simulink model "AFE_2L_H4Q"  (R2013b)
settings: Solver=FixedStepDiscrete  SolverMode=SingleTasking  StartTime=0.0  StopTime=0.9  FixedStep=Tpas  RelTol=1e-3
values from neighbouring files (symbols this model uses):
  Cbus = 330e-3    (= 0.33)    [AFE_FV_Params.m]    (also in AFE_FV_ParamsPV4.m; Params.m)
  fmod4Q = 1e3    (= 1000)    [AFE_FV_Params.m]    (also in AFE_FV_ParamsPV4.m; Params.m)
  Freq = 50    [AFE_FV_Params.m]    (also in AFE_FV_ParamsPV4.m; Params.m)
  hys = 450    [AFE_FV_Params.m]    (also in AFE_FV_ParamsPV4.m; Params.m = 300)
  I4Q = 1/0.02    (= 50)    [AFE_FV_Params.m]    (also in AFE_FV_ParamsPV4.m = (P4Q+Numd(2)/Dend(1))/Ts; CalcPIAndFilters.m = (P4Q+Numd(2)/Dend(1))/Ts; Params.m = (P4Q+Numd(2)/Dend(1))/Ts)
  Kac = 1/(Vac*sqrt(2/3))    [AFE_FV_Params.m]    (also in AFE_FV_ParamsPV4.m; Params.m)
  KLP4Q = 0.01    [AFE_FV_Params.m]    (also in AFE_FV_ParamsPV4.m = NLPripd(2); CalcPIAndFilters.m = NLPripd(2); Params.m = NLPripd(2))
  L = .1    (= 0.1)    [AFE_FV_Params.m]    (also in AFE_FV_ParamsPV4.m; Params.m)
  Lac = 8.1487e-04    (= 0.00081487)    [AFE_FV_Params.m]    (also in AFE_FV_ParamsPV4.m; Params.m)
  P4Q = 0.071    [AFE_FV_Params.m]    (also in AFE_FV_ParamsPV4.m = Numd(1)/Dend(1); CalcPIAndFilters.m = Numd(1)/Dend(1); Params.m = Numd(1)/Dend(1))
  R = .28    (= 0.28)    [AFE_FV_Params.m]    (also in AFE_FV_ParamsPV4.m; Params.m)
  SatPIH4Q = .95    (= 0.95)    [AFE_FV_Params.m]    (also in AFE_FV_ParamsPV4.m; Params.m)
  Satv = 1500    [AFE_FV_Params.m]    (also in AFE_FV_ParamsPV4.m; Params.m = 3.6e6*sqrt(2)/(sqrt(3)*Vac))
  TLP4Q = -0.99    [AFE_FV_Params.m]    (also in AFE_FV_ParamsPV4.m = DLPripd(2); CalcPIAndFilters.m = DLPripd(2); Params.m = DLPripd(2))
  Tpas = 10e-6    (= 1e-05)    [AFE_FV_Params.m]    (also in AFE_FV_ParamsPV4.m; Params.m)
  Vac = 2000    [AFE_FV_Params.m]    (also in AFE_FV_ParamsPV4.m; Params.m)
  Vdc = 5000    [AFE_FV_Params.m]    (also in AFE_FV_ParamsPV4.m; Params.m)
undefined symbols (not defined in the file or in its folder): Rac
libraries: powerlib x27, powerlib_meascontrol x17, simulink x14
settings Model: Creator=LiberT  LastModifiedBy=LiberT
settings DataIOCC: SignalLoggingSaveFormat=ModelDataLogs
settings OptimizationCC: ExpressionDepthLimit=2147483647
settings DebuggingCC: MultiTaskDSMMsg=warning  MultiTaskCondExecSysMsg=none  FcnCallInpInsideContextMsg=EnableAllAsWarning  StateNameClashWarn=warning
settings RTWCC: IncludeERTFirstTime=on

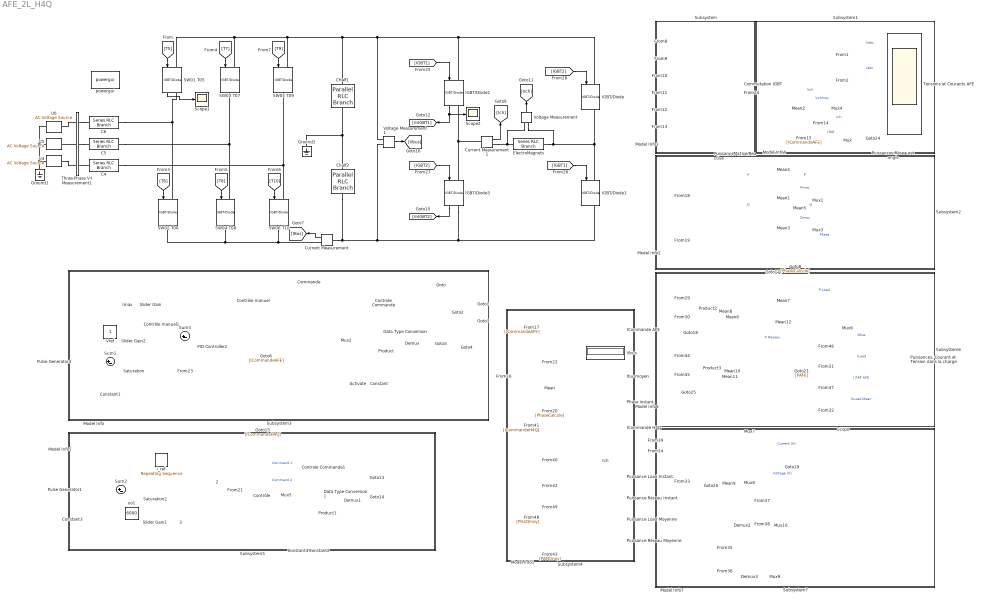
== system AFE_2L_H4Q ==
  " 2" : ManualSwitch
  " 3" : ManualSwitch  CurrentSetting=0
  Activate : Constant  Value=0
  C4 : powerlib/Elements/Series RLC Branch  LConnTagsString=__new0  RConnTagsString=__new0  BranchType=L  Resistance=Rac  Inductance=Lac  SetiL0=off  InitialCurrent=0  Capacitance=300e-3  Setx0=off  InitialVoltage=0  Measurements=None
  C5 : powerlib/Elements/Series RLC Branch  LConnTagsString=__new0  RConnTagsString=__new0  BranchType=L  Resistance=Rac  Inductance=Lac  SetiL0=off  InitialCurrent=0  Capacitance=300e-3  Setx0=off  InitialVoltage=0  Measurements=None
  C6 : powerlib/Elements/Series RLC Branch  LConnTagsString=__new0  RConnTagsString=__new0  BranchType=L  Resistance=Rac  Inductance=Lac  SetiL0=off  InitialCurrent=0  Capacitance=300e-3  Setx0=off  InitialVoltage=0  Measurements=None
  CHalf1 : powerlib/Elements/Parallel RLC Branch  LConnTagsString=a  RConnTagsString=__new0  BranchType=C  Resistance=inf  Inductance=inf  SetiL0=off  InitialCurrent=0  Capacitance=Cbus*2  Setx0=on  InitialVoltage=Vdc/2  Measurements=Branch voltage
  Chalf2 : powerlib/Elements/Parallel RLC Branch  LConnTagsString=a  RConnTagsString=__new0  BranchType=C  Resistance=inf  Inductance=inf  SetiL0=off  InitialCurrent=0  Capacitance=Cbus*2  Setx0=on  InitialVoltage=Vdc/2  Measurements=Branch voltage
  Commande : Subsystem
  Commutation IGBT : Scope  NumInputPorts=6
      settings: TickLabels=on  TimeRange=0.04  YMin=-0.2~-0.2~-0.2~-0.2~-0.2~-0.2  YMax=1.2~1.2~1.2~1.2~1.2~1.2
  Constant : Constant  Value=[1 1 1 1 1 1]
  Constant1 : Constant  Value=6000
  Constant2 : Constant  Value=[1 1]
  Constant3 : Constant  Value=6000
  Constant4 : Constant  Value=0
  Controle Commande : ManualSwitch
  Controle Commande1 : ManualSwitch
  Contrôle : Subsystem  TreatAsAtomicUnit=on
      settings: MinAlgLoopOccurrences=on
  Contrôle manuel : ManualSwitch  CurrentSetting=0
  Contrôle manuel1 : ManualSwitch
  Current Measurement : powerlib/Measurements/Current Measurement  PhasorSimulation=off  OutputType=Complex  PSBequivalent=0
  Current Measurement1 : powerlib/Measurements/Current Measurement  PhasorSimulation=off  OutputType=Complex  PSBequivalent=0
  Data Type Conversion : DataTypeConversion  OutDataTypeStr=boolean
  Data Type Conversion1 : DataTypeConversion  OutDataTypeStr=boolean
  Demux : Demux  Outputs=6
  Demux1 : Demux  Outputs=2
  Demux2 : Demux  Outputs=2
  Demux3 : Demux  Outputs=2
  "ElectroMagnets " : powerlib/Elements/Series RLC Branch  LConnTagsString=__new0  RConnTagsString=__new0  BranchType=RL  Resistance=R  Inductance=L  SetiL0=off  InitialCurrent=0  Capacitance=1e-6  Setx0=off  InitialVoltage=0  Measurements=Branch voltage and current
  Ground1 : powerlib/Elements/Ground  LConnTagsString=a
  Ground2 : powerlib/Elements/Ground  LConnTagsString=a
  "ICommande AFE " : Display
  ICommande H4Q : Display
  IGBT/Diode{,1..3} (4 alike) : powerlib/Power Electronics/IGBT//Diode  Ron=1e-3  Rs=1e5  Cs=inf  Measurements=on
  Ibusmoyen : Display
  Ich : Display
  Imax : Constant  Value=5000
  Mean{,1..3} (4 alike) : powerlib_meascontrol/Measurements/Mean  Freq=50  Vinit=0  Ts=Tpas
  Mean10 : powerlib_meascontrol/Measurements/Mean  Freq=fmod4Q/2  Vinit=0  Ts=Tpas
  Mean11 : powerlib_meascontrol/Measurements/Mean  Freq=1/.9  Vinit=0  Ts=Tpas
  Mean12 : powerlib_meascontrol/Measurements/Mean  Freq=fmod4Q  Vinit=0  Ts=Tpas
  Mean4 : powerlib_meascontrol/Measurements/Mean  Freq=fmod4Q*3  Vinit=0  Ts=Tpas
  Mean5 : powerlib_meascontrol/Measurements/Mean  Freq=fmod4Q*3  Vinit=0  Ts=Tpas
  Mean6 : powerlib_meascontrol/Measurements/Mean  Freq=1/.9  Vinit=0  Ts=Tpas
  Mean7 : powerlib_meascontrol/Measurements/Mean  Freq=fmod4Q  Vinit=0  Ts=Tpas
  Mean8 : powerlib_meascontrol/Measurements/Mean  Freq=fmod4Q/2  Vinit=0  Ts=Tpas
  Mean9 : powerlib_meascontrol/Measurements/Mean  Freq=fmod4Q  Vinit=0  Ts=Tpas
  Model Info : simulink/Model-Wide Utilities/Model Info  InitialBlockCM=None  BlockCM=None  Frame=on  DisplayStringWithTags=Commande AFE  HorizontalTextAlignment=Center  LeftAlignmentValue=0.5  SourceBlockDiagram=AFE_2L_H4Q  TagMaxNumber=20
  Model Info{1..4,6..7} (6 alike) : simulink/Model-Wide Utilities/Model Info  InitialBlockCM=None  BlockCM=None  Frame=on  DisplayStringWithTags=Résultats  HorizontalTextAlignment=Center  LeftAlignmentValue=0.5  SourceBlockDiagram=AFE_2L_H4Q  TagMaxNumber=20
  Model Info5 : simulink/Model-Wide Utilities/Model Info  InitialBlockCM=None  BlockCM=None  Frame=on  DisplayStringWithTags=Commande H4Q  HorizontalTextAlignment=Center  LeftAlignmentValue=0.5  SourceBlockDiagram=AFE_2L_H4Q  TagMaxNumber=20
  Mux{,1,3..10} (10 alike) : Mux  Inputs=2
  Mux2 : Mux  Inputs=6
  PID Controller2 : simulink/Continuous/PID Controller  Controller=PI  TimeDomain=Discrete-time  SampleTime=Tpas  IntegratorMethod=Forward Euler  FilterMethod=Forward Euler  Form=Parallel  P=150  I=1.2e4  D=0  N=100  InitialConditionSource=internal  InitialConditionForIntegrator=0  InitialConditionForFilter=0  ExternalReset=none  LimitOutput=on  UpperSaturationLimit=Satv  LowerSaturationLimit=-Satv  LinearizeAsGain=on  AntiWindupMode=clamping  Kb=1  TrackingMode=off  Kt=1  PParamMin=[]  PParamMax=[]  IParamMin=[]  IParamMax=[]  DParamMin=[]  DParamMax=[]  NParamMin=[]  NParamMax=[]  KbParamMin=[]  KbParamMax=[]  KtParamMin=[]  KtParamMax=[]  POutMin=[]  POutMax=[]  IOutMin=[]  IOutMax=[]  DOutMin=[]  DOutMax=[]  NOutMin=[]  NOutMax=[]  KbOutMin=[]  KbOutMax=[]  KtOutMin=[]  KtOutMax=[]  IntegratorOutMin=[]  IntegratorOutMax=[]  FilterOutMin=[]  FilterOutMax=[]  SumOutMin=[]  SumOutMax=[]  SumI1OutMin=[]  SumI1OutMax=[]  SumI2OutMin=[]  SumI2OutMax=[]  SumI3OutMin=[]  SumI3OutMax=[]  SumDOutMin=[]  SumDOutMax=[]  SaturationOutMin=[]  SaturationOutMax=[]  IntegratorContinuousStateAttributes=''  IntegratorStateMustResolveToSignalObject=off  IntegratorRTWStateStorageClass=Auto  FilterContinuousStateAttributes=''  FilterStateMustResolveToSignalObject=off  FilterRTWStateStorageClass=Auto
  Phase instant. : Display
  Product{,1..3} (4 alike) : Product
  Puissance Active/Reactive : Subsystem
  Puissance Load Instant. : Display
  Puissance Load Moyenne : Display
  Puissance Réseau Instant : Display
  Puissance Réseau Moyenne : Display
  Puissances Réseau et angle : Scope  NumInputPorts=3
      settings: TickLabels=on  TimeRange=0.04  YMin=-1000000~-400000~-200  YMax=10000000~350000~200  SaveName=ScopeData2
  "Puissances, Courant et Tension dans la charge" : Scope  NumInputPorts=5
      settings: TickLabels=on  ShowLegends=on  TimeRange=0.9  YMin=-20000000~3000~-1000~-3000~-5000  YMax=20000000~5250~7000~3000~5000  SaveName=ScopeData3
  Pulse Generator1 : DiscretePulseGenerator  Amplitude=12000  Period=floor(.4 /Tpas)  PulseWidth=floor(.4 * .5 / Tpas)  PhaseDelay=floor(.001 / Tpas)  SampleTime=Tpas
  Pulse Generator3 : DiscretePulseGenerator  Amplitude=12000  Period=floor(.2/Tpas)  PulseWidth=floor(.2/2/Tpas)  SampleTime=Tpas
  SW01 T05 : powerlib/Power Electronics/IGBT//Diode  Ron=1e-3  Rs=1e5  Cs=Tpas  Measurements=on
  SW02 T06 : powerlib/Power Electronics/IGBT//Diode  Ron=1e-3  Rs=1e5  Cs=Tpas  Measurements=off
  SW03 T07 : powerlib/Power Electronics/IGBT//Diode  Ron=1e-3  Rs=1e5  Cs=Tpas  Measurements=off
  SW04 T08 : powerlib/Power Electronics/IGBT//Diode  Ron=1e-3  Rs=1e5  Cs=Tpas  Measurements=off
  SW05 T09 : powerlib/Power Electronics/IGBT//Diode  Ron=1e-3  Rs=1e5  Cs=Tpas  Measurements=off
  SW06 T10 : powerlib/Power Electronics/IGBT//Diode  Ron=1e-3  Rs=1e5  Cs=Tpas  Measurements=off
  Saturation : Saturate  UpperLimit=5100  LowerLimit=5000
  Saturation2 : Saturate  UpperLimit=5000  LowerLimit=2000
  Scope : Scope  NumInputPorts=6
      settings: TimeRange=0.9  YMin=-7000~-12500~-0.1~-0.1~-7000~-6000  YMax=7000~7500~1.1~1.1~7000~6000  SaveName=hash  MaxDataPoints=10000
  Scope1 : Scope
      settings: SaveName=IGBTA
  Scope2 : Scope
      settings: SaveName=IGBTH
  Slider Gain : simulink/Math Operations/Slider Gain  low=0  gain=0.22  high=1
  Slider Gain1 : simulink/Math Operations/Slider Gain  low=0  gain=0.54  high=1
  Slider Gain2 : simulink/Math Operations/Slider Gain  low=0  gain=5000  high=6000
  Subsystem : Subsystem
      mask Display: disp('')
  Subsystem1 : Subsystem
      mask Display: disp('')
  Subsystem2 : Subsystem
      mask Display: disp('')
  Subsystem3 : Subsystem
      mask Display: disp('')
  Subsystem4 : Subsystem
      mask Display: disp('')
  Subsystem5 : Subsystem
      mask Display: disp('')
  Subsystem6 : Subsystem
      mask Display: disp('')
  Subsystem7 : Subsystem
      mask Display: disp('')
  Sum1 : Sum  Inputs=|+-
  Sum2 : Sum  Inputs=|+-
  Sum3 : Sum  Inputs=|+-
  Tensions et Courants AFE : Scope  NumInputPorts=4
      settings: TickLabels=on  ShowLegends=on  TimeRange=0.04  YMin=-1750~-2000~3000~-2000  YMax=1750~2000~5150~2000  SaveName=hach4quadrants
  Three-Phase V-I Measurement1 : powerlib/Measurements/Three-Phase V-I Measurement  VoltageMeasurement=phase-to-ground  SetLabelV=on  LabelV=Vabc  Vpu=off  VpuLL=off  CurrentMeasurement=yes  SetLabelI=on  LabelI=Iabc  Ipu=off  Pbase=100e6  Vbase=500e3  OutputType=Complex  PhasorSimulation=off  PSBequivalent=0
  U4 : powerlib/Electrical Sources/AC Voltage Source  Amplitude=Vac*sqrt(2/3)  Phase=120  Frequency=Freq  SampleTime=Tpas  Measurements=Voltage
  U5 : powerlib/Electrical Sources/AC Voltage Source  Amplitude=Vac*sqrt(2/3)  Phase=-120  Frequency=Freq  SampleTime=Tpas  Measurements=Voltage
  U6 : powerlib/Electrical Sources/AC Voltage Source  Amplitude=Vac*sqrt(2/3)  Phase=0  Frequency=Freq  SampleTime=Tpas  Measurements=Voltage
  Vbus : Display
  Voltage Measurement : powerlib/Measurements/Voltage Measurement  PhasorSimulation=off  OutputType=Complex  PSBequivalent=0
  Voltage Measurement1 : powerlib/Measurements/Voltage Measurement  PhasorSimulation=off  OutputType=Complex  PSBequivalent=0
  Vref : Constant  SampleTime=Tpas
  "i_ref " : simulink/Sources/Repeating Sequence  rep_seq_t="[0 108.51e-3 127.6e-3 132e-3 200e-3 250e-3 283.33e-3 310e-3 366.66e-3  490e-3 533e-3 683.33e-3 900e-3]"  rep_seq_y=[333 333 1000 1031 1500 2000 2500 3000 4000 6000 6000 333 333]
  powergui : powerlib/powergui  Priority=1  SimulationMode=Discrete  SolverType=Tustin  SampleTime=Tpas  frequency=60  SPID=off  DisableSnubberDevices=off  DisableRonSwitches=off  DisableVfSwitches=off  SwTol=0  Interpol=off  DisplayEquations=off  frequencyindice=50  Pbase=100e6  ErrMax=1e-4  Iterations=50  UnitsV=kV  UnitsW=MW  FunctionMessages=off  echomessages=off  HookPort=off  EnableUseOfTLC=off  x0status=blocks  RestoreLinks=warning  ResistiveCurrentMeasurement=off  Frange=[0:2:500]  Ylog=off  Xlog=on  ShowGrid=off  save=off  variable=ZData  structure=ScopeData1  ZoomFFT=off  StartTime=18  cycles=100  DisplayStyle=1  fundamental=50  FreqAxis=off  MaxFrequency=2000  frequencyindicesteady=1  RmsSteady=1  display=off  Ts=0  methode=off
  uo1 : Constant  Value=6000
  wires:
  [T5] -> SW01 T05/1
  Current Measurement/1 -> [IBus]
  [T7] -> SW03 T07/1
  [T9] -> SW05 T09/1
  [T10] -> SW06 T10/1
  [T8] -> SW04 T08/1
  [T6] -> SW02 T06/1
  [T5] -> Commutation IGBT/1
  [T6] -> Commutation IGBT/2
  [T7] -> Commutation IGBT/3
  [T8] -> Commutation IGBT/4
  [T9] -> Commutation IGBT/5
  [T10] -> Commutation IGBT/6
  [Vabc] -> Tensions et Courants AFE/1  "Vabc"
  [Iabc] -> Tensions et Courants AFE/2  "Iabc"
  Imax/1 -> Slider Gain/1
  [IBus] -> Mux/1  "Ich"
  [ICommandeAFE] -> Mux/2  "I Ref"
  Mux/1 -> [IBusScope], Tensions et Courants AFE/4
  Mean/1 -> Ibusmoyen/1
  [Vbus] -> Vbus/1
  [IBus] -> Mean/1
  [ICommandeAFE] -> "ICommande AFE "/1
  [Vbus] -> Sum3/2
  Vref/1 -> Slider Gain2/1
  Sum3/1 -> PID Controller2/1
  Constant/1 -> Product/2
  Activate/1 -> Product/1
  Commande/1(T5) -> Mux2/1
  Commande/2(T6) -> Mux2/2
  Commande/3(T7) -> Mux2/3
  Commande/4(T8) -> Mux2/4
  Commande/5(T9) -> Mux2/5
  Commande/6(T10) -> Mux2/6
  Controle Commande/1 -> Demux/1
  Mux2/1 -> Controle Commande/1
  Demux/1 -> [T5]
  Demux/2 -> [T6]
  Demux/3 -> [T7]
  Demux/4 -> [T8]
  Demux/5 -> [T9]
  Demux/6 -> [T10]
  [Vabc] -> Puissance Active/Reactive/1(Vabc)
  [Iabc] -> Puissance Active/Reactive/2(Iabc)
  Puissance Active/Reactive/1(P) -> Mean4/1, Mean1/1  "P"
  Puissance Active/Reactive/2(Q) -> Mean3/1, Mean5/1  "Q"
  Puissance Active/Reactive/3(PhC) -> Puissances Réseau et angle/3, [PhaseCalcule]  "Phase"
  Mean1/1 -> Mux1/2  "Pmoy"
  Mux1/1 -> Puissances Réseau et angle/1
  Mean3/1 -> Mux3/2  "Qmoy"
  Mux3/1 -> Puissances Réseau et angle/2
  Mux4/1 -> Tensions et Courants AFE/3
  [Vbus] -> Mux4/1, Mean2/1  "Vch"
  Mean2/1 -> Mux4/2  "Vchmoy"
  [PhaseCalcule] -> Phase instant./1
  PID Controller2/1 -> Contrôle manuel/2
  Slider Gain/1 -> Contrôle manuel/1
  Contrôle manuel/1 -> Commande/1(In1), [ICommandeAFE]
  Data Type Conversion/1 -> Controle Commande/2
  Product/1 -> Data Type Conversion/1
  Sum1/1 -> Saturation/1
  Pulse Generator3/1 -> Sum1/1
  Constant1/1 -> Sum1/2
  Contrôle manuel1/1 -> Sum3/1
  Slider Gain2/1 -> Contrôle manuel1/1
  Saturation/1 -> Contrôle manuel1/2
  IGBT/Diode2/1 -> Scope2/1, [mIGBT1]
  IGBT/Diode3/1 -> [mIGBT2]
  [IGBT1] -> IGBT/Diode2/1
  [IGBT1] -> IGBT/Diode1/1
  [IGBT2] -> IGBT/Diode3/1
  [IGBT2] -> IGBT/Diode/1
  Current Measurement1/1 -> [Ich]
  Voltage Measurement/1 -> [Vch]
  Constant2/1 -> Product1/2
  Constant4/1 -> Product1/1
  Controle Commande1/1 -> Demux1/1
  Mux5/1 -> Controle Commande1/1
  Demux1/1 -> [IGBT1]
  Demux1/2 -> [IGBT2]
  Data Type Conversion1/1 -> Controle Commande1/2
  Product1/1 -> Data Type Conversion1/1
  " 2"/1 -> [ICommandeH4Q], Contrôle/1(Iref)
  [Ich] -> Contrôle/2(IL)
  Contrôle/2(C2) -> Mux5/2  "Command 2"
  Contrôle/1(C1) -> Mux5/1  "Command 1"
  uo1/1 -> Slider Gain1/1
  Slider Gain1/1 -> " 3"/2
  Saturation2/1 -> " 3"/1
  Constant3/1 -> Sum2/2
  "i_ref "/1 -> " 2"/1
  " 3"/1 -> " 2"/2
  Pulse Generator1/1 -> Sum2/1
  Sum2/1 -> Saturation2/1
  Voltage Measurement1/1 -> [Vbus]
  Mean4/1 -> Mux1/1  "P"
  Mean5/1 -> Mux3/1  "Q"
  Mean6/1 -> [PH4Qmoy]
  [Vch] -> Product2/1
  [Ich] -> Product2/2
  Product2/1 -> Mean8/1
  Mean8/1 -> Mean6/1, Mean7/1
  Mux7/1 -> [ILoadScope], Scope/1  "Current (A)"
  Mux8/1 -> Scope/2  "Voltage (V)"
  [Ich] -> Mux7/2
  [mIGBT1] -> Demux2/1
  Mean9/1 -> [VMeanLoad], Mux8/2
  [Vch] -> Mux8/1, Mean9/1
  [mIGBT2] -> Demux3/1
  [IGBT1] -> Scope/3
  Mux9/1 -> Scope/6
  Mux10/1 -> Scope/5
  [IGBT2] -> Scope/4
  Demux2/1 -> Mux10/1
  Demux3/1 -> Mux10/2
  Demux2/2 -> Mux9/1
  Demux3/2 -> Mux9/2
  [ICommandeH4Q] -> Mux7/1
  [PAFEmoy] -> Puissance Réseau Moyenne/1
  [PH4Q] -> Puissance Load Instant./1
  [Ich] -> Ich/1
  [ICommandeH4Q] -> ICommande H4Q/1
  Mean7/1 -> [PH4Q], Mux6/1  "P Load"
  [VMeanLoad] -> "Puissances, Courant et Tension dans la charge"/5  "VLoad Mean"
  Mux6/1 -> "Puissances, Courant et Tension dans la charge"/1
  [Vbus] -> "Puissances, Courant et Tension dans la charge"/2  "VBus"
  [ILoadScope] -> "Puissances, Courant et Tension dans la charge"/3  "ILoad"
  [ICommandeAFE] -> "Puissances, Courant et Tension dans la charge"/4  "I REF AFE"
  [IBus] -> Product3/1
  [Vbus] -> Product3/2
  Product3/1 -> Mean10/1
  Mean10/1 -> Mean11/1, Mean12/1  "P Réseau"
  Mean11/1 -> [PAFEmoy]
  [PAFE] -> Puissance Réseau Instant/1
  [PH4Qmoy] -> Puissance Load Moyenne/1
  Mean12/1 -> [PAFE], Mux6/2
  SW01 T05/1 -> Scope1/1
  connections:
  Current Measurement/RConn1 -- SW06 T10/RConn1 -- SW04 T08/RConn1 -- SW02 T06/RConn1
  SW02 T06/LConn1 -- C6/LConn1 -- SW01 T05/RConn1
  SW06 T10/LConn1 -- C4/LConn1 -- SW05 T09/RConn1
  SW04 T08/LConn1 -- C5/LConn1 -- SW03 T07/RConn1
  Three-Phase V-I Measurement1/LConn1 -- C6/RConn1
  Three-Phase V-I Measurement1/RConn1 -- U6/RConn1
  Three-Phase V-I Measurement1/RConn2 -- U5/RConn1
  Three-Phase V-I Measurement1/LConn2 -- C5/RConn1
  C4/RConn1 -- Three-Phase V-I Measurement1/LConn3
  U4/RConn1 -- Three-Phase V-I Measurement1/RConn3
  IGBT/Diode3/RConn1 -- Voltage Measurement1/LConn2 -- Chalf2/RConn1 -- Current Measurement/LConn1 -- IGBT/Diode1/RConn1
  U4/LConn1 -- U6/LConn1 -- U5/LConn1 -- Ground1/LConn1
  Chalf2/LConn1 -- Ground2/LConn1 -- CHalf1/RConn1
  IGBT/Diode3/LConn1 -- Current Measurement1/LConn1 -- IGBT/Diode2/RConn1
  SW01 T05/LConn1 -- Voltage Measurement1/LConn1 -- IGBT/Diode2/LConn1 -- IGBT/Diode/LConn1 -- CHalf1/LConn1 -- SW05 T09/LConn1 -- SW03 T07/LConn1
  "ElectroMagnets "/RConn1 -- Voltage Measurement/LConn2 -- IGBT/Diode1/LConn1 -- IGBT/Diode/RConn1
  Current Measurement1/RConn1 -- Voltage Measurement/LConn1 -- "ElectroMagnets "/LConn1

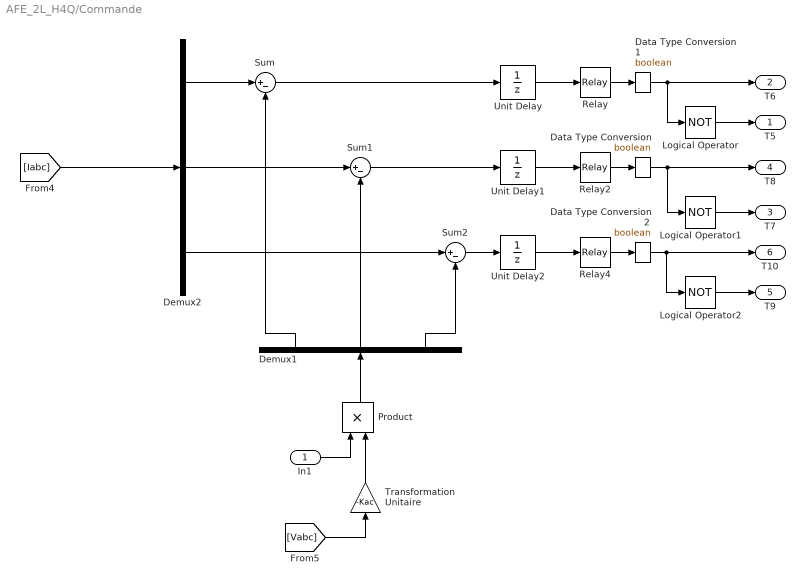
== system AFE_2L_H4Q/Commande ==
  In1 : Inport
  Data Type Conversion : DataTypeConversion  OutDataTypeStr=boolean
  Data Type Conversion1 : DataTypeConversion  OutDataTypeStr=boolean
  Data Type Conversion2 : DataTypeConversion  OutDataTypeStr=boolean
  Demux1 : Demux  Outputs=3
  Demux2 : Demux  Outputs=3
  Logical Operator : Logic  Operator=NOT  AllPortsSameDT=off
  Logical Operator1 : Logic  Operator=NOT  AllPortsSameDT=off
  Logical Operator2 : Logic  Operator=NOT  AllPortsSameDT=off
  Product : Product
  Relay : Relay  OnSwitchValue=hys  OffSwitchValue=-hys
  Relay2 : Relay  OnSwitchValue=hys  OffSwitchValue=-hys
  Relay4 : Relay  OnSwitchValue=hys  OffSwitchValue=-hys
  Sum : Sum  Inputs=|+-
  Sum1 : Sum  Inputs=|+-
  Sum2 : Sum  Inputs=|+-
  Transformation Unitaire : Gain  Gain=-Kac
  Unit Delay : UnitDelay  SampleTime=-1
  Unit Delay1 : UnitDelay  SampleTime=-1
  Unit Delay2 : UnitDelay  SampleTime=-1
  T5 : Outport
  T6 : Outport  Port=2
  T7 : Outport  Port=3
  T8 : Outport  Port=4
  T9 : Outport  Port=5
  T10 : Outport  Port=6
  wires:
  Demux2/1 -> Sum/1
  Demux2/2 -> Sum1/1
  Demux2/3 -> Sum2/1
  Sum/1 -> Unit Delay/1
  Sum1/1 -> Unit Delay1/1
  Sum2/1 -> Unit Delay2/1
  Unit Delay/1 -> Relay/1
  Unit Delay1/1 -> Relay2/1
  Unit Delay2/1 -> Relay4/1
  Logical Operator/1 -> T5/1
  Logical Operator1/1 -> T7/1
  Logical Operator2/1 -> T9/1
  Relay/1 -> Data Type Conversion1/1
  Relay2/1 -> Data Type Conversion/1
  Relay4/1 -> Data Type Conversion2/1
  [Iabc] -> Demux2/1
  [Vabc] -> Transformation Unitaire/1
  Demux1/1 -> Sum/2
  Demux1/2 -> Sum1/2
  Demux1/3 -> Sum2/2
  Data Type Conversion/1 -> T8/1, Logical Operator1/1
  Data Type Conversion1/1 -> T6/1, Logical Operator/1
  Data Type Conversion2/1 -> T10/1, Logical Operator2/1
  Transformation Unitaire/1 -> Product/2
  In1/1 -> Product/1
  Product/1 -> Demux1/1

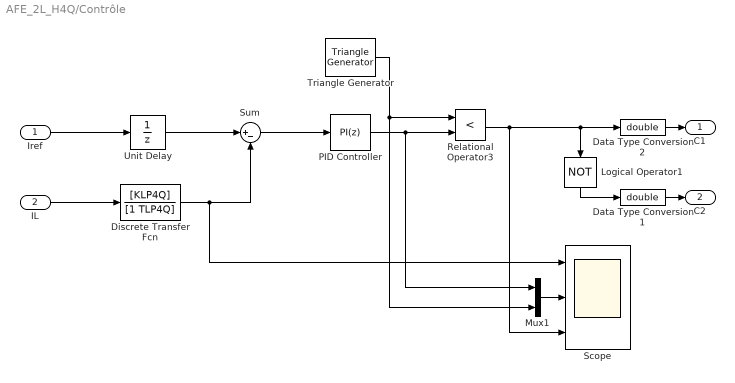
== system AFE_2L_H4Q/Contrôle ==
  Iref : Inport
  IL : Inport  Port=2
  Data Type Conversion1 : DataTypeConversion  OutDataTypeStr=double
  Data Type Conversion2 : DataTypeConversion  OutDataTypeStr=double
  Discrete Transfer Fcn : DiscreteTransferFcn  Numerator=[KLP4Q]  Denominator=[1 TLP4Q]
  Logical Operator1 : Logic  Operator=NOT  AllPortsSameDT=off  OutDataTypeStr=boolean
  Mux1 : Mux  Inputs=2
  PID Controller : simulink/Continuous/PID Controller  Controller=PI  TimeDomain=Discrete-time  SampleTime=Tpas  IntegratorMethod=Forward Euler  FilterMethod=Forward Euler  Form=Parallel  P=P4Q  I=I4Q  D=0  N=100  InitialConditionSource=internal  InitialConditionForIntegrator=0  InitialConditionForFilter=0  ExternalReset=none  LimitOutput=on  UpperSaturationLimit=SatPIH4Q  LowerSaturationLimit=-SatPIH4Q  LinearizeAsGain=on  AntiWindupMode=clamping  Kb=1  TrackingMode=off  Kt=1  PParamMin=[]  PParamMax=[]  IParamMin=[]  IParamMax=[]  DParamMin=[]  DParamMax=[]  NParamMin=[]  NParamMax=[]  KbParamMin=[]  KbParamMax=[]  KtParamMin=[]  KtParamMax=[]  POutMin=[]  POutMax=[]  IOutMin=[]  IOutMax=[]  DOutMin=[]  DOutMax=[]  NOutMin=[]  NOutMax=[]  KbOutMin=[]  KbOutMax=[]  KtOutMin=[]  KtOutMax=[]  IntegratorOutMin=[]  IntegratorOutMax=[]  FilterOutMin=[]  FilterOutMax=[]  SumOutMin=[]  SumOutMax=[]  SumI1OutMin=[]  SumI1OutMax=[]  SumI2OutMin=[]  SumI2OutMax=[]  SumI3OutMin=[]  SumI3OutMax=[]  SumDOutMin=[]  SumDOutMax=[]  SaturationOutMin=[]  SaturationOutMax=[]  IntegratorContinuousStateAttributes=''  IntegratorStateMustResolveToSignalObject=off  IntegratorRTWStateStorageClass=Auto  FilterContinuousStateAttributes=''  FilterStateMustResolveToSignalObject=off  FilterRTWStateStorageClass=Auto
  Relational Operator3 : RelationalOperator  Operator=<  OutDataTypeStr=boolean
  Scope : Scope  NumInputPorts=3
      settings: TimeRange=0.01  YMin=0~-1.2~-5  YMax=6000~1.2~5
  Sum : Sum  Inputs=|+-
  Triangle Generator : powerlib_meascontrol/Pulse & Signal Generators/Triangle Generator  Freq=fmod4Q  Phase=180  Ts=Tpas
  Unit Delay : UnitDelay  SampleTime=-1
  C1 : Outport
  C2 : Outport  Port=2
  wires:
  Triangle Generator/1 -> Mux1/2, Relational Operator3/1
  Relational Operator3/1 -> Logical Operator1/1, Data Type Conversion2/1, Scope/3
  Data Type Conversion2/1 -> C1/1
  Logical Operator1/1 -> Data Type Conversion1/1
  Data Type Conversion1/1 -> C2/1
  Discrete Transfer Fcn/1 -> Scope/1, Sum/2
  Mux1/1 -> Scope/2
  PID Controller/1 -> Relational Operator3/2, Mux1/1
  Sum/1 -> PID Controller/1
  IL/1 -> Discrete Transfer Fcn/1
  Iref/1 -> Unit Delay/1
  Unit Delay/1 -> Sum/1

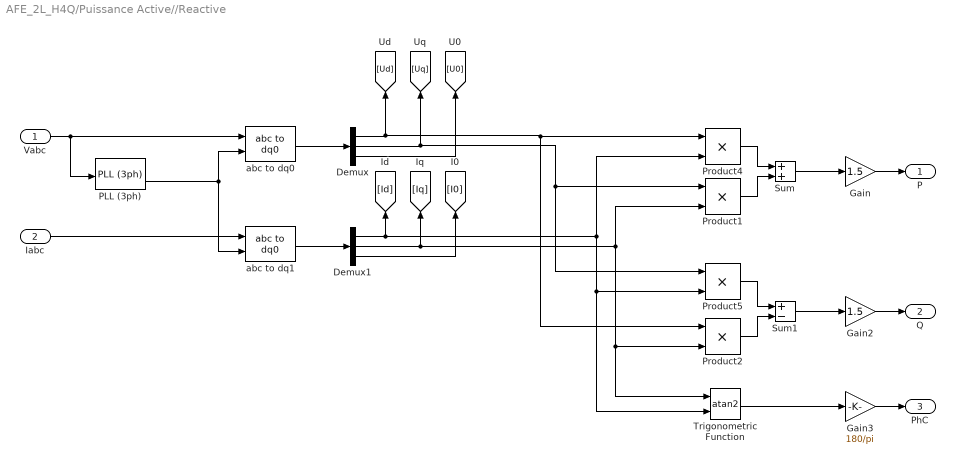
== system AFE_2L_H4Q/Puissance Active//Reactive ==
  Vabc : Inport
  Iabc : Inport  Port=2
  Demux : Demux  Outputs=3
  Demux1 : Demux  Outputs=3
  Gain : Gain  Gain=1.5
  Gain2 : Gain  Gain=1.5
  Gain3 : Gain  Gain=180/pi
  PLL (3ph) : powerlib_meascontrol/PLL/PLL (3ph)  Fmin=49  Par_Init=[0, 50]  ParK=[180, 3200, 1]  TcD=1e-4  MaxRateChangeFreq=6  FilterCutOffFreq=25  Ts=Tpas  AGC=on
  Product{1..2,4..5} (4 alike) : Product
  Sum : Sum
  Sum1 : Sum  Inputs=+-
  Trigonometric Function : Trigonometry  Operator=atan2
  abc to dq0 : powerlib_meascontrol/Transformations/abc to dq0  Alignment=90 degrees behind phase A axis
  abc to dq1 : powerlib_meascontrol/Transformations/abc to dq0  Alignment=90 degrees behind phase A axis
  P : Outport
  Q : Outport  Port=2
  PhC : Outport  Port=3
  wires:
  Vabc/1 -> PLL (3ph)/1, abc to dq0/1
  abc to dq0/1 -> Demux/1
  abc to dq1/1 -> Demux1/1
  Product2/1 -> Sum1/2
  Sum1/1 -> Gain2/1
  Demux/3 -> [U0]
  Demux/2 -> Product5/1, Product1/1, [Uq]
  Demux/1 -> Product2/1, Product4/1, [Ud]
  Demux1/2 -> [Iq], Trigonometric Function/1, Product2/2, Product1/2
  Product5/1 -> Sum1/1
  Gain2/1 -> Q/1
  Trigonometric Function/1 -> Gain3/1
  Gain3/1 -> PhC/1
  Product4/1 -> Sum/1
  Product1/1 -> Sum/2
  Sum/1 -> Gain/1
  Gain/1 -> P/1
  Demux1/1 -> [Id], Trigonometric Function/2, Product5/2, Product4/2
  Demux1/3 -> [I0]
  PLL (3ph)/2 -> abc to dq1/2, abc to dq0/2
  Iabc/1 -> abc to dq1/1

== system AFE_2L_H4Q/Subsystem ==

== system AFE_2L_H4Q/Subsystem1 ==

== system AFE_2L_H4Q/Subsystem2 ==

== system AFE_2L_H4Q/Subsystem3 ==

== system AFE_2L_H4Q/Subsystem4 ==

== system AFE_2L_H4Q/Subsystem5 ==

== system AFE_2L_H4Q/Subsystem6 ==

== system AFE_2L_H4Q/Subsystem7 ==
